simulink model "untitled_2"  (Simulink 8.3)
settings: Solver=ode45  StartTime=0.0  StopTime=10.0  RelTol=1e-3
settings Model: Creator=Радион  LastModifiedBy=Радион
settings OptimizationCC: BooleanDataType=off
settings DebuggingCC: SaveWithParameterizedLinksMsg=none  SignalResolutionControl=TryResolveAllWithWarning  SolverPrmCheckMsg=none  MultiTaskDSMMsg=warning  MultiTaskCondExecSysMsg=none  StateNameClashWarn=none
settings HardwareCC: TargetUnknown=on
settings RTWCC: IncludeERTFirstTime=on

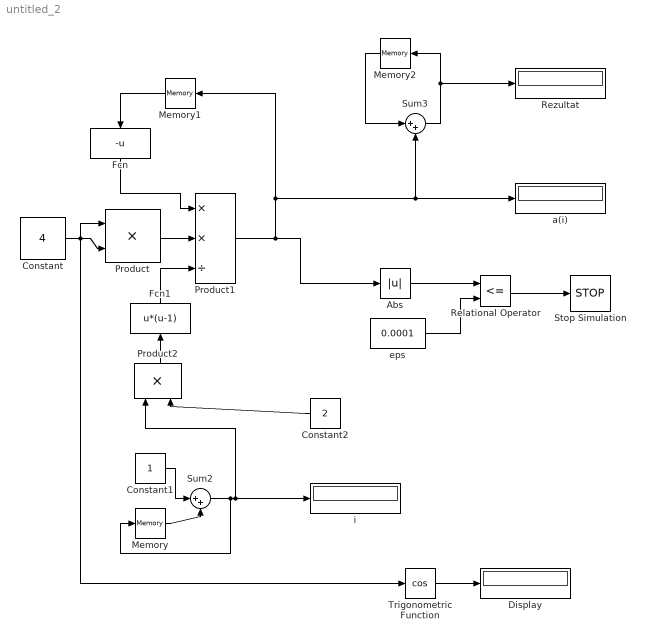
== system untitled_2 ==
  Abs : Abs  SaturateOnIntegerOverflow=on
  Constant : Constant  Value=4  VectorParams1D=off
  Constant1 : Constant
  Constant2 : Constant  Value=2
  Display : Display
  Fcn : Fcn  Expr=-u
  Fcn1 : Fcn  Expr=u*(u-1)
  Memory : Memory
  Memory1 : Memory  X0=1
  Memory2 : Memory  X0=1
  Product : Product  SaturateOnIntegerOverflow=on  RndMeth=Zero  InputSameDT=on  OutDataTypeStr=Inherit: Same as first input
  Product1 : Product  Inputs=**/  SaturateOnIntegerOverflow=on  RndMeth=Zero  InputSameDT=on  OutDataTypeStr=Inherit: Same as first input
  Product2 : Product  SaturateOnIntegerOverflow=on  RndMeth=Zero  InputSameDT=on  OutDataTypeStr=Inherit: Same as first input
  Relational Operator : RelationalOperator  Operator=<=  InputSameDT=on
  Rezultat : Display
  Stop Simulation : Stop
  Sum2 : Sum  Inputs=|++  SaturateOnIntegerOverflow=on  InputSameDT=on  OutDataTypeStr=Inherit: Same as first input
  Sum3 : Sum  Inputs=|++  SaturateOnIntegerOverflow=on  InputSameDT=on  OutDataTypeStr=Inherit: Same as first input
  Trigonometric Function : Trigonometry  Operator=cos
  a(i) : Display
  eps : Constant  Value=0.0001  VectorParams1D=off
  i : Display
  wires:
  Constant/1 -> Trigonometric Function/1, Product/1, Product/2
  Trigonometric Function/1 -> Display/1
  Product/1 -> Product1/2
  Constant1/1 -> Sum2/1
  Sum2/1 -> Memory/1, i/1, Product2/1
  Product1/1 -> Abs/1, Memory1/1, a(i)/1, Sum3/2
  Abs/1 -> Relational Operator/1
  eps/1 -> Relational Operator/2
  Relational Operator/1 -> Stop Simulation/1
  Fcn/1 -> Product1/1
  Sum3/1 -> Memory2/1, Rezultat/1
  Memory2/1 -> Sum3/1
  Memory1/1 -> Fcn/1
  Constant2/1 -> Product2/2
  Memory/1 -> Sum2/2
  Product2/1 -> Fcn1/1
  Fcn1/1 -> Product1/3
